simulink model "LKAS_SIL"  (R2018b)
settings: Solver=FixedStepDiscrete  StartTime=0.0  StopTime=90  FixedStep=0.01  MaxStep=0.01  RelTol=1e-3
model workspace (MAT data in the model file):
  LKA_CarWidth = Simulink.Parameter
  LKA_CarWidth.Value = 1.8
  LKA_CarWidth.DataType = 'single'
  LKA_CarWidth.Dimensions = [1 1]
  LKA_SampleTime = Simulink.Parameter
  LKA_SampleTime.Value = 0.01
  LKA_SampleTime.DataType = 'single'
  LKA_SampleTime.Dimensions = [1 1]
  LKA_StrRatio_C = Simulink.Parameter
  LKA_StrRatio_C.Value = 15.3
  LKA_StrRatio_C.DataType = 'single'
  LKA_StrRatio_C.Dimensions = [1 1]
  LKA_Veh2CamL_C = Simulink.Parameter
  LKA_Veh2CamL_C.Value = 1.56
  LKA_Veh2CamL_C.DataType = 'single'
  LKA_Veh2CamL_C.Dimensions = [1 1]
  LKA_Veh2CamW_C = Simulink.Parameter
  LKA_Veh2CamW_C.Value = 0.9
  LKA_Veh2CamW_C.DataType = 'single'
  LKA_Veh2CamW_C.Dimensions = [1 1]
  LKA_WhlBaseL_C = Simulink.Parameter
  LKA_WhlBaseL_C.Value = 2.65
  LKA_WhlBaseL_C.DataType = 'single'
  LKA_WhlBaseL_C.Dimensions = [1 1]
  LL_CompSWA_C = Simulink.Parameter
  LL_CompSWA_C.Value = 0
  LL_CompSWA_C.DataType = 'single'
  LL_CompSWA_C.Dimensions = [1 1]
  LL_CrvtPrvwT_C = Simulink.Parameter
  LL_CrvtPrvwT_C.Value = 0.45
  LL_CrvtPrvwT_C.DataType = 'single'
  LL_CrvtPrvwT_C.Dimensions = [1 1]
  LL_DesDvt_C = Simulink.Parameter
  LL_DesDvt_C.Value = 0.2
  LL_DesDvt_C.DataType = 'single'
  LL_DesDvt_C.Dimensions = [1 1]
  LL_DvtComp_C = Simulink.Parameter
  LL_DvtComp_C.Value = 0
  LL_DvtComp_C.DataType = 'single'
  LL_DvtComp_C.Dimensions = [1 1]
  LL_DvtPrvwT_C = Simulink.Parameter
  LL_DvtPrvwT_C.Value = 0.45
  LL_DvtPrvwT_C.DataType = 'single'
  LL_DvtPrvwT_C.Dimensions = [1 1]
  LL_DvtSpdDet_vDvtSpdMin_C = Simulink.Parameter
  LL_DvtSpdDet_vDvtSpdMin_C.Value = 0
  LL_DvtSpdDet_vDvtSpdMin_C.DataType = 'single'
  LL_DvtSpdDet_vDvtSpdMin_C.Dimensions = [1 1]
  LL_HdAgExT_C = Simulink.Parameter
  LL_HdAgExT_C.Value = 15
  LL_HdAgExT_C.DataType = 'single'
  LL_HdAgExT_C.Dimensions = [1 1]
  LL_HdAgPrvwT_C = Simulink.Parameter
  LL_HdAgPrvwT_C.Value = 0.45
  LL_HdAgPrvwT_C.DataType = 'single'
  LL_HdAgPrvwT_C.Dimensions = [1 1]
  LL_LAccMax_C = Simulink.Parameter
  LL_LAccMax_C.Value = 3
  LL_LAccMax_C.DataType = 'single'
  LL_LAccMax_C.Dimensions = [1 1]
  LL_LAccRMax_C = Simulink.Parameter
  LL_LAccRMax_C.Value = 5
  LL_LAccRMax_C.DataType = 'single'
  LL_LAccRMax_C.Dimensions = [1 1]
  LL_LDWS_SUPPRESS_HEADING = Simulink.Parameter
  LL_LDWS_SUPPRESS_HEADING.Value = 2
  LL_LDWS_SUPPRESS_HEADING.DataType = 'single'
  LL_LDWS_SUPPRESS_HEADING.Dimensions = [1 1]
  LL_LDW_EarliestWarnLine_C = Simulink.Parameter
  LL_LDW_EarliestWarnLine_C.Value = 0.3
  LL_LDW_EarliestWarnLine_C.DataType = 'single'
  LL_LDW_EarliestWarnLine_C.Dimensions = [1 1]
  LL_LDW_LatestWarnLine_C = Simulink.Parameter
  LL_LDW_LatestWarnLine_C.Value = -0.4
  LL_LDW_LatestWarnLine_C.DataType = 'single'
  LL_LDW_LatestWarnLine_C.Dimensions = [1 1]
  LL_LFClb_TFC_DiffCtlBalance = Simulink.Parameter
  LL_LFClb_TFC_DiffCtlBalance.Value = 0
  LL_LFClb_TFC_DiffCtlBalance.DataType = 'single'
  LL_LFClb_TFC_DiffCtlBalance.Dimensions = [1 1]
  LL_LFClb_TFC_DiffCtrlMaxSWA = Simulink.Parameter
  LL_LFClb_TFC_DiffCtrlMaxSWA.Value = 20
  LL_LFClb_TFC_DiffCtrlMaxSWA.DataType = 'single'
  LL_LFClb_TFC_DiffCtrlMaxSWA.Dimensions = [1 1]
  LL_LFClb_TFC_DiffCtrlRatio = Simulink.Parameter
  LL_LFClb_TFC_DiffCtrlRatio.Value = 400
  LL_LFClb_TFC_DiffCtrlRatio.DataType = 'single'
  LL_LFClb_TFC_DiffCtrlRatio.Dimensions = [1 1]
  LL_LFClb_TFC_FfCtlRatio_C = Simulink.Parameter
  LL_LFClb_TFC_FfCtlRatio_C.Value = 1
  LL_LFClb_TFC_FfCtlRatio_C.DataType = 'single'
  LL_LFClb_TFC_FfCtlRatio_C.Dimensions = [1 1]
  LL_LFClb_TFC_facmGainLutGain1_C = Simulink.Parameter
  LL_LFClb_TFC_facmGainLutGain1_C.Value = 40
  LL_LFClb_TFC_facmGainLutGain1_C.DataType = 'single'
  LL_LFClb_TFC_facmGainLutGain1_C.Dimensions = [1 1]
  LL_LFClb_TFC_facmGainLutGain2_C = Simulink.Parameter
  LL_LFClb_TFC_facmGainLutGain2_C.Value = 40
  LL_LFClb_TFC_facmGainLutGain2_C.DataType = 'single'
  LL_LFClb_TFC_facmGainLutGain2_C.Dimensions = [1 1]
  LL_LFClb_TFC_facmIntegRatio = Simulink.Parameter
  LL_LFClb_TFC_facmIntegRatio.Value = 0.002
  LL_LFClb_TFC_facmIntegRatio.DataType = 'single'
  LL_LFClb_TFC_facmIntegRatio.Dimensions = [1 1]
  LL_LFClb_TFC_facmKlat_C = Simulink.Parameter
  LL_LFClb_TFC_facmKlat_C.Value = -9
  LL_LFClb_TFC_facmKlat_C.DataType = 'single'
  LL_LFClb_TFC_facmKlat_C.Dimensions = [1 1]
  LL_LFClb_TFC_phiIntegCtlMaxSWA_C = Simulink.Parameter
  LL_LFClb_TFC_phiIntegCtlMaxSWA_C.Value = 5
  LL_LFClb_TFC_phiIntegCtlMaxSWA_C.DataType = 'single'
  LL_LFClb_TFC_phiIntegCtlMaxSWA_C.Dimensions = [1 1]
  LL_LFClb_TFC_tiKlatPrvwT_C = Simulink.Parameter
  LL_LFClb_TFC_tiKlatPrvwT_C.Value = 2
  LL_LFClb_TFC_tiKlatPrvwT_C.DataType = 'single'
  LL_LFClb_TFC_tiKlatPrvwT_C.Dimensions = [1 1]
  LL_LFClb_TFC_vGainLutVehSpdLwr_C = Simulink.Parameter
  LL_LFClb_TFC_vGainLutVehSpdLwr_C.Value = 60
  LL_LFClb_TFC_vGainLutVehSpdLwr_C.DataType = 'single'
  LL_LFClb_TFC_vGainLutVehSpdLwr_C.Dimensions = [1 1]
  LL_LFClb_TFC_vGainLutVehSpdUpr_C = Simulink.Parameter
  LL_LFClb_TFC_vGainLutVehSpdUpr_C.Value = 120
  LL_LFClb_TFC_vGainLutVehSpdUpr_C.DataType = 'single'
  LL_LFClb_TFC_vGainLutVehSpdUpr_C.Dimensions = [1 1]
  LL_LKAExPrcs_ExitC0Dvt = Simulink.Parameter
  LL_LKAExPrcs_ExitC0Dvt.Value = 0.01
  LL_LKAExPrcs_ExitC0Dvt.DataType = 'single'
  LL_LKAExPrcs_ExitC0Dvt.Dimensions = [1 1]
  LL_LKAExPrcs_ExitC0Swt = Simulink.Parameter
  LL_LKAExPrcs_ExitC0Swt.Value = 1
  LL_LKAExPrcs_ExitC0Swt.DataType = 'single'
  LL_LKAExPrcs_ExitC0Swt.Dimensions = [1 1]
  LL_LKAExPrcs_tiExitTime1 = Simulink.Parameter
  LL_LKAExPrcs_tiExitTime1.Value = 8
  LL_LKAExPrcs_tiExitTime1.DataType = 'single'
  LL_LKAExPrcs_tiExitTime1.Dimensions = [1 1]
  LL_LKAExPrcs_tiExitTime2 = Simulink.Parameter
  LL_LKAExPrcs_tiExitTime2.Value = 4
  LL_LKAExPrcs_tiExitTime2.DataType = 'single'
  LL_LKAExPrcs_tiExitTime2.Dimensions = [1 1]
  LL_LKAExPrcs_tiExitTime3 = Simulink.Parameter
  LL_LKAExPrcs_tiExitTime3.Value = 0.2
  LL_LKAExPrcs_tiExitTime3.DataType = 'single'
  LL_LKAExPrcs_tiExitTime3.Dimensions = [1 1]
  LL_LKASWASyn_M0 = Simulink.Parameter
  LL_LKASWASyn_M0.Value = 0.4
  LL_LKASWASyn_M0.DataType = 'single'
  LL_LKASWASyn_M0.Dimensions = [1 1]
  LL_LKASWASyn_M1 = Simulink.Parameter
  LL_LKASWASyn_M1.Value = 0.8
  LL_LKASWASyn_M1.DataType = 'single'
  LL_LKASWASyn_M1.Dimensions = [1 1]
  LL_LKASWASyn_M2 = Simulink.Parameter
  LL_LKASWASyn_M2.Value = 0.3
  LL_LKASWASyn_M2.DataType = 'single'
  LL_LKASWASyn_M2.Dimensions = [1 1]
  LL_LKASWASyn_M3K = Simulink.Parameter
  LL_LKASWASyn_M3K.Value = 0.2
  LL_LKASWASyn_M3K.DataType = 'single'
  LL_LKASWASyn_M3K.Dimensions = [1 1]
  LL_LKASWASyn_SWAaddMax = Simulink.Parameter
  LL_LKASWASyn_SWAaddMax.Value = 8
  LL_LKASWASyn_SWAaddMax.DataType = 'single'
  LL_LKASWASyn_SWAaddMax.Dimensions = [1 1]
  LL_LKASWASyn_T2 = Simulink.Parameter
  LL_LKASWASyn_T2.Value = 4
  LL_LKASWASyn_T2.DataType = 'single'
  LL_LKASWASyn_T2.Dimensions = [1 1]
  LL_LKASWASyn_TrqMax = Simulink.Parameter
  LL_LKASWASyn_TrqMax.Value = 1.5
  LL_LKASWASyn_TrqMax.DataType = 'single'
  LL_LKASWASyn_TrqMax.Dimensions = [1 1]
  LL_LKASWASyn_TrqSwaAddSwt = Simulink.Parameter
  LL_LKASWASyn_TrqSwaAddSwt.Value = 0
  LL_LKASWASyn_TrqSwaAddSwt.DataType = 'single'
  LL_LKASWASyn_TrqSwaAddSwt.Dimensions = [1 1]
  LL_LKASWASyn_TrqSwaRateDiff = Simulink.Parameter
  LL_LKASWASyn_TrqSwaRateDiff.Value = -0.2
  LL_LKASWASyn_TrqSwaRateDiff.DataType = 'single'
  LL_LKASWASyn_TrqSwaRateDiff.Dimensions = [1 1]
  LL_LKASWASyn_tiTrqSwaRtTime = Simulink.Parameter
  LL_LKASWASyn_tiTrqSwaRtTime.Value = 0.2
  LL_LKASWASyn_tiTrqSwaRtTime.DataType = 'single'
  LL_LKASWASyn_tiTrqSwaRtTime.Dimensions = [1 1]
  LL_LKASWASyn_tiTrqSwaTime = Simulink.Parameter
  LL_LKASWASyn_tiTrqSwaTime.Value = 0.3
  LL_LKASWASyn_tiTrqSwaTime.DataType = 'single'
  LL_LKASWASyn_tiTrqSwaTime.Dimensions = [1 1]
  LL_LKAS_OUT_OF_CONTROL_LAT_VEL = Simulink.Parameter
  LL_LKAS_OUT_OF_CONTROL_LAT_VEL.Value = 1.5
  LL_LKAS_OUT_OF_CONTROL_LAT_VEL.DataType = 'single'
  LL_LKAS_OUT_OF_CONTROL_LAT_VEL.Dimensions = [1 1]
  LL_LKAS_OUT_OF_CONTROL_TTLC = Simulink.Parameter
  LL_LKAS_OUT_OF_CONTROL_TTLC.Value = 0.3
  LL_LKAS_OUT_OF_CONTROL_TTLC.DataType = 'single'
  LL_LKAS_OUT_OF_CONTROL_TTLC.Dimensions = [1 1]
  LL_LKA_EarliestWarnLine_C = Simulink.Parameter
  LL_LKA_EarliestWarnLine_C.Value = 0.3
  LL_LKA_EarliestWarnLine_C.DataType = 'single'
  LL_LKA_EarliestWarnLine_C.Dimensions = [1 1]
  LL_LKA_LatestWarnLine_C = Simulink.Parameter
  LL_LKA_LatestWarnLine_C.Value = -0.5
  LL_LKA_LatestWarnLine_C.DataType = 'single'
  LL_LKA_LatestWarnLine_C.Dimensions = [1 1]
  LL_LSpdCompT_C = Simulink.Parameter
  LL_LSpdCompT_C.Value = 0.4
  LL_LSpdCompT_C.DataType = 'single'
  LL_LSpdCompT_C.Dimensions = [1 1]
  LL_MAX_DELAY_EPSSTAR_TIME = Simulink.Parameter
  LL_MAX_DELAY_EPSSTAR_TIME.Value = 0.5
  LL_MAX_DELAY_EPSSTAR_TIME.DataType = 'single'
  LL_MAX_DELAY_EPSSTAR_TIME.Dimensions = [1 1]
  LL_MAX_DRIVER_TORQUE_DISABLE = Simulink.Parameter
  LL_MAX_DRIVER_TORQUE_DISABLE.Value = 2.25
  LL_MAX_DRIVER_TORQUE_DISABLE.DataType = 'single'
  LL_MAX_DRIVER_TORQUE_DISABLE.Dimensions = [1 1]
  LL_MAX_DRIVER_TORQUE_ENABLE = Simulink.Parameter
  LL_MAX_DRIVER_TORQUE_ENABLE.Value = 3
  LL_MAX_DRIVER_TORQUE_ENABLE.DataType = 'single'
  LL_MAX_DRIVER_TORQUE_ENABLE.Dimensions = [1 1]
  LL_MAX_LANE_WIDTH_DISABLE = Simulink.Parameter
  LL_MAX_LANE_WIDTH_DISABLE.Value = 5.5
  LL_MAX_LANE_WIDTH_DISABLE.DataType = 'single'
  LL_MAX_LANE_WIDTH_DISABLE.Dimensions = [1 1]
  LL_MAX_LANE_WIDTH_ENABLE = Simulink.Parameter
  LL_MAX_LANE_WIDTH_ENABLE.Value = 5.4
  LL_MAX_LANE_WIDTH_ENABLE.DataType = 'single'
  LL_MAX_LANE_WIDTH_ENABLE.Dimensions = [1 1]
  LL_MAX_LAT_ACC_DISABLE = Simulink.Parameter
  LL_MAX_LAT_ACC_DISABLE.Value = 3.5
  LL_MAX_LAT_ACC_DISABLE.DataType = 'single'
  LL_MAX_LAT_ACC_DISABLE.Dimensions = [1 1]
  LL_MAX_LAT_ACC_ENABLE = Simulink.Parameter
  LL_MAX_LAT_ACC_ENABLE.Value = 3
  LL_MAX_LAT_ACC_ENABLE.DataType = 'single'
  LL_MAX_LAT_ACC_ENABLE.Dimensions = [1 1]
  LL_MAX_LDWS_SPEED_DISABLE = Simulink.Parameter
  LL_MAX_LDWS_SPEED_DISABLE.Value = 150
  LL_MAX_LDWS_SPEED_DISABLE.DataType = 'single'
  LL_MAX_LDWS_SPEED_DISABLE.Dimensions = [1 1]
  LL_MAX_LDWS_SPEED_ENABLE = Simulink.Parameter
  LL_MAX_LDWS_SPEED_ENABLE.Value = 140
  LL_MAX_LDWS_SPEED_ENABLE.DataType = 'single'
  LL_MAX_LDWS_SPEED_ENABLE.Dimensions = [1 1]
  LL_MAX_LKAS_SPEED_DISABLE = Simulink.Parameter
  LL_MAX_LKAS_SPEED_DISABLE.Value = 150
  LL_MAX_LKAS_SPEED_DISABLE.DataType = 'single'
  LL_MAX_LKAS_SPEED_DISABLE.Dimensions = [1 1]
  LL_MAX_LKAS_SPEED_ENABLE = Simulink.Parameter
  LL_MAX_LKAS_SPEED_ENABLE.Value = 140
  LL_MAX_LKAS_SPEED_ENABLE.DataType = 'single'
  LL_MAX_LKAS_SPEED_ENABLE.Dimensions = [1 1]
  LL_MAX_LONG_ACC_DISABLE = Simulink.Parameter
  LL_MAX_LONG_ACC_DISABLE.Value = 3.5
  LL_MAX_LONG_ACC_DISABLE.DataType = 'single'
  LL_MAX_LONG_ACC_DISABLE.Dimensions = [1 1]
  LL_MAX_LONG_ACC_ENABLE = Simulink.Parameter
  LL_MAX_LONG_ACC_ENABLE.Value = 3
  LL_MAX_LONG_ACC_ENABLE.DataType = 'single'
  LL_MAX_LONG_ACC_ENABLE.Dimensions = [1 1]
  LL_MAX_LONG_DECEL_DISABLE = Simulink.Parameter
  LL_MAX_LONG_DECEL_DISABLE.Value = 2.5
  LL_MAX_LONG_DECEL_DISABLE.DataType = 'single'
  LL_MAX_LONG_DECEL_DISABLE.Dimensions = [1 1]
  LL_MAX_LONG_DECEL_ENABLE = Simulink.Parameter
  LL_MAX_LONG_DECEL_ENABLE.Value = 2
  LL_MAX_LONG_DECEL_ENABLE.DataType = 'single'
  LL_MAX_LONG_DECEL_ENABLE.Dimensions = [1 1]
  LL_MAX_STEER_ANGLE_DISABLE = Simulink.Parameter
  LL_MAX_STEER_ANGLE_DISABLE.Value = 70
  LL_MAX_STEER_ANGLE_DISABLE.DataType = 'single'
  LL_MAX_STEER_ANGLE_DISABLE.Dimensions = [1 1]
  LL_MAX_STEER_ANGLE_ENABLE = Simulink.Parameter
  LL_MAX_STEER_ANGLE_ENABLE.Value = 60
  LL_MAX_STEER_ANGLE_ENABLE.DataType = 'single'
  LL_MAX_STEER_ANGLE_ENABLE.Dimensions = [1 1]
  LL_MAX_STEER_SPEED_DISABLE = Simulink.Parameter
  LL_MAX_STEER_SPEED_DISABLE.Value = 5000
  LL_MAX_STEER_SPEED_DISABLE.DataType = 'single'
  LL_MAX_STEER_SPEED_DISABLE.Dimensions = [1 1]
  LL_MAX_STEER_SPEED_ENABLE = Simulink.Parameter
  LL_MAX_STEER_SPEED_ENABLE.Value = 5000
  LL_MAX_STEER_SPEED_ENABLE.DataType = 'single'
  LL_MAX_STEER_SPEED_ENABLE.Dimensions = [1 1]
  LL_MAX_SYSTEM_CURVATURE_DISABLE = Simulink.Parameter
  LL_MAX_SYSTEM_CURVATURE_DISABLE.Value = 0.0055
  LL_MAX_SYSTEM_CURVATURE_DISABLE.DataType = 'single'
  LL_MAX_SYSTEM_CURVATURE_DISABLE.Dimensions = [1 1]
  LL_MAX_SYSTEM_CURVATURE_ENABLE = Simulink.Parameter
  LL_MAX_SYSTEM_CURVATURE_ENABLE.Value = 0.0045
  LL_MAX_SYSTEM_CURVATURE_ENABLE.DataType = 'single'
  LL_MAX_SYSTEM_CURVATURE_ENABLE.Dimensions = [1 1]
  LL_MIN_LANE_WIDTH_DISABLE = Simulink.Parameter
  LL_MIN_LANE_WIDTH_DISABLE.Value = 2.4
  LL_MIN_LANE_WIDTH_DISABLE.DataType = 'single'
  LL_MIN_LANE_WIDTH_DISABLE.Dimensions = [1 1]
  LL_MIN_LANE_WIDTH_ENABLE = Simulink.Parameter
  LL_MIN_LANE_WIDTH_ENABLE.Value = 2.5
  LL_MIN_LANE_WIDTH_ENABLE.DataType = 'single'
  LL_MIN_LANE_WIDTH_ENABLE.Dimensions = [1 1]
  LL_MIN_LKAS_SPEED_DISABLE = Simulink.Parameter
  LL_MIN_LKAS_SPEED_DISABLE.Value = 55
  LL_MIN_LKAS_SPEED_DISABLE.DataType = 'single'
  LL_MIN_LKAS_SPEED_DISABLE.Dimensions = [1 1]
  LL_MIN_LKAS_SPEED_ENABLE = Simulink.Parameter
  LL_MIN_LKAS_SPEED_ENABLE.Value = 60
  LL_MIN_LKAS_SPEED_ENABLE.DataType = 'single'
  LL_MIN_LKAS_SPEED_ENABLE.Dimensions = [1 1]
  LL_Max_LDWS_Warning_Time = Simulink.Parameter
  LL_Max_LDWS_Warning_Time.Value = 5
  LL_Max_LDWS_Warning_Time.DataType = 'single'
  LL_Max_LDWS_Warning_Time.Dimensions = [1 1]
  LL_NomTAhd_C = Simulink.Parameter
  LL_NomTAhd_C.Value = 0.2
  LL_NomTAhd_C.DataType = 'single'
  LL_NomTAhd_C.Dimensions = [1 1]
  LL_ThresDet_lDvtThresLwrLDW = Simulink.Parameter
  LL_ThresDet_lDvtThresLwrLDW.Value = 0.15
  LL_ThresDet_lDvtThresLwrLDW.DataType = 'single'
  LL_ThresDet_lDvtThresLwrLDW.Dimensions = [1 1]
  LL_ThresDet_lDvtThresLwrLKA = Simulink.Parameter
  LL_ThresDet_lDvtThresLwrLKA.Value = 0.3
  LL_ThresDet_lDvtThresLwrLKA.DataType = 'single'
  LL_ThresDet_lDvtThresLwrLKA.Dimensions = [1 1]
  LL_ThresDet_lDvtThresUprLDW = Simulink.Parameter
  LL_ThresDet_lDvtThresUprLDW.Value = 0.3
  LL_ThresDet_lDvtThresUprLDW.DataType = 'single'
  LL_ThresDet_lDvtThresUprLDW.Dimensions = [1 1]
  LL_ThresDet_lDvtThresUprLKA = Simulink.Parameter
  LL_ThresDet_lDvtThresUprLKA.Value = 0.6
  LL_ThresDet_lDvtThresUprLKA.DataType = 'single'
  LL_ThresDet_lDvtThresUprLKA.Dimensions = [1 1]
  LL_ThresDet_tiTTLCThresLDW = Simulink.Parameter
  LL_ThresDet_tiTTLCThresLDW.Value = 0.75
  LL_ThresDet_tiTTLCThresLDW.DataType = 'single'
  LL_ThresDet_tiTTLCThresLDW.Dimensions = [1 1]
  LL_ThresDet_tiTTLCThresLKA = Simulink.Parameter
  LL_ThresDet_tiTTLCThresLKA.Value = 1.5
  LL_ThresDet_tiTTLCThresLKA.DataType = 'single'
  LL_ThresDet_tiTTLCThresLKA.Dimensions = [1 1]
  LL_TkOvStChk_tiTDelTime = Simulink.Parameter
  LL_TkOvStChk_tiTDelTime.Value = 2
  LL_TkOvStChk_tiTDelTime.DataType = 'single'
  LL_TkOvStChk_tiTDelTime.Dimensions = [1 1]
  LL_TkOvStChk_tiTrqChkT = Simulink.Parameter
  LL_TkOvStChk_tiTrqChkT.Value = 0.1
  LL_TkOvStChk_tiTrqChkT.DataType = 'single'
  LL_TkOvStChk_tiTrqChkT.Dimensions = [1 1]
  LL_lStpLngth_C = Simulink.Parameter
  LL_lStpLngth_C.Value = 5
  LL_lStpLngth_C.DataType = 'single'
  LL_lStpLngth_C.Dimensions = [1 1]
  ob_LKA_Version = Simulink.Signal
  ob_LKA_Version.DataType = 'single'
  ob_LKA_Version.Dimensions = -1
  ob_LKA_Version.DimensionsMode = 'auto'
  ob_LKA_Version.Complexity = 'auto'
  ob_LKA_Version.SampleTime = -1
  ob_LKA_Version.SamplingMode = 'auto'
undefined symbols (not defined in the file or in its folder): LKA_CarWidth, LKA_SampleTime, LKA_StrRatio_C, LKA_Veh2CamL_C, LKA_Veh2CamW_C, LKA_WhlBaseL_C, LL_CompSWA_C, LL_CrvtPrvwT_C, LL_DesDvt_C, LL_DvtComp_C, LL_DvtPrvwT_C, LL_DvtSpdDet_vDvtSpdMin_C, LL_HdAgExT_C, LL_HdAgPrvwT_C, LL_LAccMax_C, LL_LAccRMax_C, LL_LDW_EarliestWarnLine_C, LL_LDW_LatestWarnLine_C, LL_LDWS_SUPPRESS_HEADING, LL_LFClb_TFC_DiffCtlBalance, LL_LFClb_TFC_DiffCtrlMaxSWA, LL_LFClb_TFC_DiffCtrlRatio, LL_LFClb_TFC_facmGainLutGain1_C, LL_LFClb_TFC_facmGainLutGain2_C, LL_LFClb_TFC_facmIntegRatio, LL_LFClb_TFC_facmKlat_C, LL_LFClb_TFC_FfCtlRatio_C, LL_LFClb_TFC_phiIntegCtlMaxSWA_C, LL_LFClb_TFC_tiKlatPrvwT_C, LL_LFClb_TFC_vGainLutVehSpdLwr_C, LL_LFClb_TFC_vGainLutVehSpdUpr_C, LL_LKA_EarliestWarnLine_C, LL_LKA_LatestWarnLine_C, LL_LKAExPrcs_ExitC0Dvt, LL_LKAExPrcs_ExitC0Swt, LL_LKAExPrcs_tiExitTime1, LL_LKAExPrcs_tiExitTime2, LL_LKAExPrcs_tiExitTime3, LL_LKAS_OUT_OF_CONTROL_LAT_VEL, LL_LKAS_OUT_OF_CONTROL_TTLC, LL_LKASWASyn_M0, LL_LKASWASyn_M1, LL_LKASWASyn_M2, LL_LKASWASyn_M3K, LL_LKASWASyn_SWAaddMax, LL_LKASWASyn_T2, LL_LKASWASyn_tiTrqSwaRtTime, LL_LKASWASyn_tiTrqSwaTime, LL_LKASWASyn_TrqMax, LL_LKASWASyn_TrqSwaAddSwt, LL_LKASWASyn_TrqSwaRateDiff, LL_LSpdCompT_C, LL_lStpLngth_C, LL_MAX_DELAY_EPSSTAR_TIME, LL_MAX_DRIVER_TORQUE_DISABLE, LL_MAX_DRIVER_TORQUE_ENABLE, LL_MAX_LANE_WIDTH_DISABLE, LL_MAX_LANE_WIDTH_ENABLE, LL_MAX_LAT_ACC_DISABLE, LL_MAX_LAT_ACC_ENABLE ... (+29)
libraries: simulink x134, dspstat3 x3, simulink_extras x1
(part 1 of 13)
settings Model: SimulationMode=software-in-the-loop (sil)  Creator=hejr  LastModifiedBy=hejr
settings DataIOCC: ExternalInput=[Time,GW_550_PSA1__LKA_main_switch,GW_550_PSA1__LC_Mode,EPS_495_PSA1__State_of_EPS_for_LKA_function,EPS_495_PSA1__Steering_wheel_torque,ESC_3CD_PSA1__Lateral_acceleration,ESC_3CD_PSA1__Yaw_speed,ESC_38D_PSA1__Vehicle_speed_of_wheelsensor,GW_32D_PSA1__ACCEL_LONGI_CALIB,ESC_3CD_PSA1__TMC_pressure,EPS_305_PSA1__Steering_wheel_angle,EPS_305_PSA1__Steering_wheel_rotation_speed,GW_452_PSA1__BCM_Status_Indicator,GW_349_PSA1__TCU_Gear_lever_position,Video_Lane_Left_A__C3_5FA,Video_Lane_Left_A__C2_5FA,Video_Lane_Left_A__C1_5FA,Video_Lane_Left_A__C0_5FA,Video_Lane_Left_A__Quality_5FA,Video_Lane_Left_A__Line_Type_5FA,Video_Lane_Left_B__View_Range_5FC,Video_Lane_Left_B__TLC_5FC,Video_Lane_Right_A__C3_5FD,Video_Lane_Right_A__C2_5FD,Video_Lane_Right_A__C1_5FD,Video_Lane_Right_A__C0_5FD,Video_Lane_Right_A__Quality_5FD,Video_Lane_Right_A__Line_Type_5FD,Video_Lane_Right_B__View_Range_5FF,Video_Lane_Right_B__TLC_5FF,Video_Lane_Left_A__C0_5FA,Video_Lane_Left_A__C1_5FA,Video_Lane_Left_A__C2_5FA,Video_Lane_Left_A__C3_5FA,Video_Lane_Left_B__View_Range_5FC,Video_Lane_Left_A__Quality_5FA,Video_Lane_Left_A__Line_Type_5FA,Video_Lane_Left_B__TLC_5FC,Video_Lane_Right_A__C0_5FD,Video_Lane_Right_A__C1_5FD,Video_Lane_Right_A__C2_5FD,Video_Lane_Right_A__C3_5FD,Video_Lane_Right_B__View_Range_5FF,Video_Lane_Right_A__Quality_5FD,Video_Lane_Right_A__Line_Type_5FD,Video_Lane_Right_B__TLC_5FF,ADAS_541_PSA1__LDW_Flag,ADAS_541_PSA1__Vehicle_Lane_Display,ADAS_3F2_PSA1__Column_angle_setpoint3F2,ADAS_3F2_PSA1__Permit_to_know_if_LKA_or_LPA3F2]  LoadExternalInput=on  SaveFormat=StructureWithTime  SaveOutput=off  SignalLoggingName=logsOut
settings OptimizationCC: DefaultParameterBehavior=Inlined  DefaultUnderspecifiedDataType=single  EnhancedBackFolding=on  PassReuseOutputArgsAs=Individual arguments  ZeroExternalMemoryAtStartup=off  ZeroInternalMemoryAtStartup=off  OptimizeBlockOrder=speed  DifferentSizesBufferReuse=on  OptimizationCustomize=off
settings DebuggingCC: ParameterTunabilityLossMsg=error
settings SFSimCC: MATLABDynamicMemAlloc=off
settings RTWCC: SystemTargetFile=autosar.tlc  TemplateMakefile=ert_default_tmf  Description=AUTOSAR  GenerateReport=on  Toolchain=MinGW64 | gmake (64-bit Windows)  IncludeHyperlinkInReport=on  LaunchReport=on  GenerateTraceInfo=on  GenerateTraceReport=on  GenerateTraceReportSl=on  GenerateTraceReportSf=on  GenerateTraceReportEml=on
settings CodeAppCC: ForceParamTrailComments=on  IgnoreCustomStorageClasses=off  OperatorAnnotations=on  SimulinkDataObjDesc=on  SFDataObjDesc=on  InsertBlockDesc=on
settings STFCustomTargetCC: TargetLangStandard=C99 (ISO)  MultiwordLength=256  ParMdlRefBuildCompliant=on  CompOptLevelCompliant=on  IncludeMdlTerminateFcn=off  CombineOutputUpdateFcns=on  SuppressErrorStatus=on  ERTCustomFileBanners=on  SupportNonFinite=off  SupportComplex=off  SupportContinuousTime=off  SupportNonInlinedSFcns=off  RemoveResetFunc=on  MATLABClassNameForMDSCustomization=Simulink.SoftwareTarget.ERTCustomization  AutosarCompliant=on  UseToolchainInfoCompliant=on  LookupTableObjectStructAxisOrder=2,1,3,4,...  LUTObjectStructOrderEvenSpacing=Size,Table,Breakpoints  SystemTargetFile=autosar.tlc
settings ERTTargetCC: TargetLangStandard=C99 (ISO)  ConcurrentExecutionCompliant=off  IncludeMdlTerminateFcn=off  SuppressErrorStatus=on  SupportNonFinite=off  SupportComplex=off  ModelStepFunctionPrototypeControlCompliant=off  CPPClassGenCompliant=off  AutosarCompliant=on  LookupTableObjectStructAxisOrder=2,1,3,4,...  LUTObjectStructOrderEvenSpacing=Size,Table,Breakpoints  InlinedParameterPlacement=NonHierarchical  ERTCustomFileTemplate=example_file_process.tlc

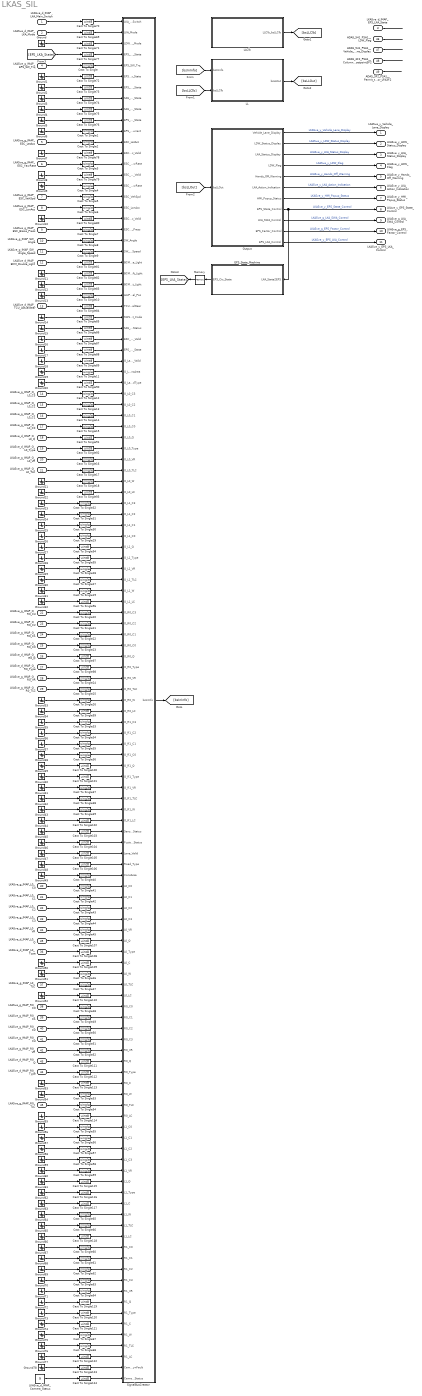
== system LKAS_SIL ==
  LKASve_d_IMAP_LKA_Main_Switch : Inport  OutDataTypeStr=double
  LKASve_d_IMAP_LKA_Mode : Inport  Port=2  OutDataTypeStr=double
  LKASve_d_IMAP_EPS_LKA_State : Inport  Port=3  OutDataTypeStr=double
  LKASve_g_IMAP_EPS_SW_Trq : Inport  Port=4  OutDataTypeStr=double
  LKASve_g_IMAP_ESC_LatAcc : Inport  Port=5  OutDataTypeStr=double
  LKASve_g_IMAP_ESC_YawRate : Inport  Port=6  OutDataTypeStr=double
  LKASve_g_IMAP_ESC_VehSpd : Inport  Port=7  OutDataTypeStr=double
  LKASve_g_IMAP_ESC_LonAcc : Inport  Port=8  OutDataTypeStr=double
  LKASve_g_IMAP_ESC_Brake_Press : Inport  Port=9  OutDataTypeStr=double
  LKASve_g_IMAP_SW_Angle : Inport  Port=10  OutDataTypeStr=double
  LKASve_g_IMAP_SW_Angle_Speed : Inport  Port=11  OutDataTypeStr=double
  LKASve_d_IMAP_BCM_Double_Light : Inport  Port=12  OutDataTypeStr=double
  LKASve_d_IMAP_TCU_ActualGear : Inport  Port=13  OutDataTypeStr=double
  LKASve_g_IMAP_O_L0_C3 : Inport  Port=14  OutDataTypeStr=double
  LKASve_g_IMAP_O_L0_C2 : Inport  Port=15  OutDataTypeStr=double
  LKASve_g_IMAP_O_L0_C1 : Inport  Port=16  OutDataTypeStr=double
  LKASve_g_IMAP_O_L0_C0 : Inport  Port=17  OutDataTypeStr=double
  LKASve_d_IMAP_O_L0_Q : Inport  Port=18  OutDataTypeStr=double
  LKASve_d_IMAP_O_L0_Type : Inport  Port=19  OutDataTypeStr=double
  LKASve_g_IMAP_O_L0_VR : Inport  Port=20  OutDataTypeStr=double
  LKASve_g_IMAP_O_L0_TLC : Inport  Port=21  OutDataTypeStr=double
  LKASve_g_IMAP_O_R0_C3 : Inport  Port=22  OutDataTypeStr=double
  LKASve_g_IMAP_O_R0_C2 : Inport  Port=23  OutDataTypeStr=double
  LKASve_g_IMAP_O_R0_C1 : Inport  Port=24  OutDataTypeStr=double
  LKASve_g_IMAP_O_R0_C0 : Inport  Port=25  OutDataTypeStr=double
  LKASve_d_IMAP_O_R0_Q : Inport  Port=26  OutDataTypeStr=double
  LKASve_d_IMAP_O_R0_Type : Inport  Port=27  OutDataTypeStr=double
  LKASve_g_IMAP_O_R0_VR : Inport  Port=28  OutDataTypeStr=double
  LKASve_g_IMAP_O_R0_TLC : Inport  Port=29  OutDataTypeStr=double
  LKASve_g_IMAP_L0_C0 : Inport  Port=30  OutDataTypeStr=double
  LKASve_g_IMAP_L0_C1 : Inport  Port=31  OutDataTypeStr=double
  LKASve_g_IMAP_L0_C2 : Inport  Port=32  OutDataTypeStr=double
  LKASve_g_IMAP_L0_C3 : Inport  Port=33  OutDataTypeStr=double
  LKASve_g_IMAP_L0_VR : Inport  Port=34  OutDataTypeStr=double
  LKASve_d_IMAP_L0_Q : Inport  Port=35  OutDataTypeStr=double
  LKASve_d_IMAP_L0_Type : Inport  Port=36  OutDataTypeStr=double
  LKASve_g_IMAP_L0_TLC : Inport  Port=37  OutDataTypeStr=double
  LKASve_g_IMAP_R0_C0 : Inport  Port=38  OutDataTypeStr=double
  LKASve_g_IMAP_R0_C1 : Inport  Port=39  OutDataTypeStr=double
  LKASve_g_IMAP_R0_C2 : Inport  Port=40  OutDataTypeStr=double
  LKASve_g_IMAP_R0_C3 : Inport  Port=41  OutDataTypeStr=double
  LKASve_g_IMAP_R0_VR : Inport  Port=42  OutDataTypeStr=double
  LKASve_d_IMAP_R0_Q : Inport  Port=43  OutDataTypeStr=double
  LKASve_d_IMAP_R0_Type : Inport  Port=44  OutDataTypeStr=double
  LKASve_g_IMAP_R0_TLC : Inport  Port=45  OutDataTypeStr=double
  ADAS_541_PSA1__LDW_Flag : Inport  Port=46  OutDataTypeStr=double
  ADAS_541_PSA1__Vehicle_Lane_Display : Inport  Port=47  OutDataTypeStr=double
  ADAS_3F2_PSA1__Column_angle_setpoint3F2 : Inport  Port=48  OutDataTypeStr=double
  ADAS_3F2_PSA1__Permit_to_know_if_LKA_or_LPA3F2 : Inport  Port=49  OutDataTypeStr=double
  Cast To Single{,1..68} (69 alike) : DataTypeConversion  OutDataTypeStr=single
  Cast To Single{69..124} (56 alike) : DataTypeConversion  OutDataTypeStr=uint8
  EPS_State_Mashine : Subsystem
  Ground{,1..78} (79 alike) : Ground
  LKASve_d_IMAP_Camera_Status : Constant  Value=9  OutDataTypeStr=uint8
  LL : Subsystem  TreatAsAtomicUnit=on
  LLClb : Subsystem
  Memory : Memory
  Output : Subsystem
  SignalBusCreator : Subsystem
  LKASve_y_Vehicle_Lane_Display : Outport
  LKASve_y_LDW_Status_Display : Outport  Port=2  SignalName=LKASve_y_LDW_Status_Display
  LKASve_y_LKA_Status_Display : Outport  Port=3
  LKASve_y_LDW_Flag : Outport  Port=4
  LKASve_y_Hands_Off_Warning : Outport  Port=5
  LKASve_y_LKA_Action_Indication : Outport  Port=6
  LKASve_y_HMI_Popup_Status : Outport  Port=7
  LKAve_y_EPS_State_Control : Outport  Port=8
  LKASve_g_LKA_SWA_Control : Outport  Port=9
  LKASve_g_EPS_Factor_Control : Outport  Port=10
  LKASve_y_EPS_LKA_Control : Outport  Port=11
  wires:
  LKASve_g_IMAP_O_L0_C1/1 -> Cast To Single14/1
  LKASve_g_IMAP_O_L0_TLC/1 -> Cast To Single17/1
  Ground61/1 -> Cast To Single115/1
  Cast To Single4/1 -> SignalBusCreator/16(ESC_UnYawRate)
  LKASve_d_IMAP_O_L0_Type/1 -> Cast To Single92/1
  Cast To Single107/1 -> SignalBusCreator/85(L0_Q)
  Cast To Single16/1 -> SignalBusCreator/41(O_L0_VR)
  Cast To Single73/1 -> SignalBusCreator/7(EPS_Trq_State)
  Cast To Single34/1 -> SignalBusCreator/66(O_R1_C2)
  Cast To Single80/1 -> SignalBusCreator/19(ESC_LonAcc_Valid)
  Ground31/1 -> Cast To Single19/1
  Cast To Single22/1 -> SignalBusCreator/57(O_R0_C1)
  Cast To Single77/1 -> SignalBusCreator/4(EPS_LKA_State)
  Cast To Single60/1 -> SignalBusCreator/113(R1_C0)
  Ground70/1 -> Cast To Single63/1
  Ground75/1 -> Cast To Single67/1
  Cast To Single49/1 -> SignalBusCreator/92(R0_C1)
  Cast To Single57/1 -> SignalBusCreator/104(L1_C2)
  Ground53/1 -> Cast To Single113/1
  LLClb/1(LLClb_bsLLClb) -> [bsLLClb]
  Ground23/1 -> Cast To Single32/1
  Cast To Single102/1 -> SignalBusCreator/74(O_R1_LC)
  Ground62/1 -> Cast To Single116/1
  Ground43/1 -> Cast To Single39/1
  Ground69/1 -> Cast To Single62/1
  LKASve_g_IMAP_L0_C0/1 -> Cast To Single41/1
  Cast To Single15/1 -> SignalBusCreator/38(O_L0_C0)
  Ground13/1 -> Cast To Single10/1
  LKASve_d_IMAP_TCU_ActualGear/1 -> Cast To Single84/1
  Cast To Single79/1 -> SignalBusCreator/15(ESC_YawRate_Valid)
  Cast To Single95/1 -> SignalBusCreator/50(O_L1_Type)
  Cast To Single99/1 -> SignalBusCreator/64(O_R0_LC)
  Cast To Single13/1 -> SignalBusCreator/36(O_L0_C2)
  LKASve_g_IMAP_SW_Angle_Speed/1 -> Cast To Single9/1
  Ground33/1 -> Cast To Single26/1
  Ground63/1 -> Cast To Single117/1
  Cast To Single45/1 -> SignalBusCreator/84(L0_VR)
  Cast To Single98/1 -> SignalBusCreator/60(O_R0_Type)
  [bsInInfo] -> LL/1(bsInInfo)
  Cast To Single113/1 -> SignalBusCreator/98(R0_C)
  Cast To Single91/1 -> SignalBusCreator/39(O_L0_Q)
  Ground24/1 -> Cast To Single31/1
  Cast To Single54/1 -> SignalBusCreator/100(R0_TLC)
  Ground48/1 -> Cast To Single106/1
  LKASve_g_IMAP_O_R0_VR/1 -> Cast To Single24/1
  LKASve_g_IMAP_O_L0_C3/1 -> Cast To Single12/1
  EPS_State_Mashine/1(EPS_Ctr_State) -> Memory/1
  Cast To Single116/1 -> SignalBusCreator/108(L1_Type)
  Cast To Single123/1 -> SignalBusCreator/124(CameraSynFault)
  LKASve_g_IMAP_SW_Angle/1 -> Cast To Single8/1
  Cast To Single124/1 -> SignalBusCreator/125(Camera_Status)
  Memory/1 -> [EPS_LKA_State]
  Cast To Single26/1 -> SignalBusCreator/63(O_R0_W)
  Cast To Single117/1 -> SignalBusCreator/109(L1_C)
  Cast To Single/1 -> SignalBusCreator/5(EPS_SW_Trq)
  Cast To Single104/1 -> SignalBusCreator/76(Fusion_Status)
  Ground20/1 -> Cast To Single90/1
  Ground35/1 -> Cast To Single33/1
  Cast To Single111/1 -> SignalBusCreator/96(R0_Q)
  Ground60/1 -> Cast To Single59/1
  Cast To Single28/1 -> SignalBusCreator/51(O_L1_VR)
  Ground7/1 -> Cast To Single78/1
  Cast To Single32/1 -> SignalBusCreator/45(O_L1_C3)
  Ground6/1 -> Cast To Single1/1
  Cast To Single109/1 -> SignalBusCreator/87(L0_C)
  Ground42/1 -> Cast To Single38/1
  LKASve_g_IMAP_O_L0_VR/1 -> Cast To Single16/1
  Cast To Single62/1 -> SignalBusCreator/115(R1_C2)
  Cast To Single64/1 -> SignalBusCreator/117(R1_VR)
  LKASve_d_IMAP_BCM_Double_Light/1 -> Cast To Single81/1
  LKASve_g_IMAP_R0_C2/1 -> Cast To Single50/1
  Cast To Single59/1 -> SignalBusCreator/106(L1_VR)
  Cast To Single37/1 -> SignalBusCreator/71(O_R1_VR)
  Cast To Single92/1 -> SignalBusCreator/40(O_L0_Type)
  LKASve_g_IMAP_L0_VR/1 -> Cast To Single45/1
  Ground5/1 -> Cast To Single76/1
  Ground51/1 -> Cast To Single46/1
  Ground32/1 -> Cast To Single96/1
  LKASve_d_IMAP_L0_Q/1 -> Cast To Single107/1
  Cast To Single122/1 -> SignalBusCreator/123(R1_LC)
  LKASve_g_IMAP_R0_C3/1 -> Cast To Single51/1
  Cast To Single58/1 -> SignalBusCreator/105(L1_C3)
  Cast To Single20/1 -> SignalBusCreator/55(O_R0_C3)
  Cast To Single118/1 -> SignalBusCreator/112(L1_LC)
  Cast To Single6/1 -> SignalBusCreator/18(ESC_LonAcc)
  LKASve_d_IMAP_R0_Type/1 -> Cast To Single112/1
  LKASve_g_IMAP_ESC_YawRate/1 -> Cast To Single3/1
  Cast To Single86/1 -> SignalBusCreator/29(SAS_In_Status)
  Ground1/1 -> Cast To Single72/1
  Cast To Single30/1 -> SignalBusCreator/47(O_L1_C1)
  Cast To Single94/1 -> SignalBusCreator/49(O_L1_Q)
  Cast To Single63/1 -> SignalBusCreator/116(R1_C3)
  Cast To Single8/1 -> SignalBusCreator/21(SW_Angle)
  Cast To Single47/1 -> SignalBusCreator/89(L0_TLC)
  Cast To Single69/1 -> SignalBusCreator/2(LKA_Mode)
  LKASve_d_IMAP_Camera_Status/1 -> Cast To Single124/1
  Cast To Single29/1 -> SignalBusCreator/48(O_L1_C0)
  LKASve_d_IMAP_EPS_LKA_State/1 -> ?
  ADAS_541_PSA1__LDW_Flag/1 -> ?
  ADAS_541_PSA1__Vehicle_Lane_Display/1 -> ?
  ADAS_3F2_PSA1__Column_angle_setpoint3F2/1 -> ?
  LKASve_g_IMAP_L0_C3/1 -> Cast To Single44/1
  Ground38/1 -> Cast To Single36/1
  Cast To Single53/1 -> SignalBusCreator/99(R0_W)
  Ground52/1 -> Cast To Single110/1
  Cast To Single97/1 -> SignalBusCreator/59(O_R0_Q)
  LKASve_g_IMAP_O_L0_C0/1 -> Cast To Single15/1
  LKASve_g_IMAP_O_R0_C2/1 -> Cast To Single21/1
  LKASve_g_IMAP_ESC_Brake_Press/1 -> Cast To Single7/1
  Cast To Single101/1 -> SignalBusCreator/70(O_R1_Type)
  Cast To Single48/1 -> SignalBusCreator/91(R0_C0)
  LKASve_g_IMAP_ESC_VehSpd/1 -> Cast To Single5/1
  Cast To Single67/1 -> SignalBusCreator/121(R1_W)
  Ground39/1 -> Cast To Single100/1
  Cast To Single93/1 -> SignalBusCreator/44(O_L0_LC)
  Ground21/1 -> Cast To Single18/1
  Cast To Single83/1 -> SignalBusCreator/25(BCM_Right_Light)
  Cast To Single74/1 -> SignalBusCreator/8(SAS_Clb_State)
  Cast To Single121/1 -> SignalBusCreator/120(R1_C)
  Ground71/1 -> Cast To Single64/1
  Cast To Single36/1 -> SignalBusCreator/68(O_R1_C0)
  Cast To Single40/1 -> SignalBusCreator/79(ConsArea)
  Cast To Single12/1 -> SignalBusCreator/35(O_L0_C3)
  SignalBusCreator/1(bsInInfo) -> [bsInInfo]
  Ground30/1 -> Cast To Single27/1
  Ground16/1 -> Cast To Single87/1
  Ground8/1 -> Cast To Single79/1
  Cast To Single50/1 -> SignalBusCreator/93(R0_C2)
  Ground74/1 -> Cast To Single121/1
  Ground3/1 -> Cast To Single74/1
  Cast To Single1/1 -> SignalBusCreator/11(EPS_LKA_Current)
  LKASve_d_IMAP_O_R0_Type/1 -> Cast To Single98/1
  Cast To Single7/1 -> SignalBusCreator/20(ESC_Brake_Press)
  Ground12/1 -> Cast To Single83/1
  LKASve_g_IMAP_L0_C2/1 -> Cast To Single43/1
  Cast To Single105/1 -> SignalBusCreator/77(Lane_Valid)
  Ground18/1 -> Cast To Single89/1
  [EPS_LKA_State] -> Cast To Single77/1
  LKASve_g_IMAP_L0_TLC/1 -> Cast To Single47/1
  LKASve_g_IMAP_O_L0_C2/1 -> Cast To Single13/1
  Cast To Single71/1 -> SignalBusCreator/3(LDW_Warn_Mode)
  Cast To Single66/1 -> SignalBusCreator/111(L1_TLC)
  Ground66/1 -> Cast To Single118/1
  LKASve_g_IMAP_ESC_LonAcc/1 -> Cast To Single6/1
  LKASve_d_IMAP_O_R0_Q/1 -> Cast To Single97/1
  Ground64/1 -> Cast To Single65/1
  Ground37/1 -> Cast To Single35/1
  Cast To Single55/1 -> SignalBusCreator/102(L1_C0)
  Cast To Single120/1 -> SignalBusCreator/119(R1_Type)
  Cast To Single112/1 -> SignalBusCreator/97(R0_Type)
  Cast To Single115/1 -> SignalBusCreator/107(L1_Q)
  Cast To Single110/1 -> SignalBusCreator/90(L0_LC)
  ADAS_3F2_PSA1__Permit_to_know_if_LKA_or_LPA3F2/1 -> ?
  Cast To Single27/1 -> SignalBusCreator/52(O_L1_TLC)
  Cast To Single119/1 -> SignalBusCreator/118(R1_Q)
  Ground/1 -> Cast To Single71/1
  Cast To Single44/1 -> SignalBusCreator/83(L0_C3)
  Ground14/1 -> Cast To Single85/1
  LKASve_g_IMAP_R0_C1/1 -> Cast To Single49/1
  Cast To Single87/1 -> SignalBusCreator/30(ESC_VehSpd_Valid)
  Cast To Single75/1 -> SignalBusCreator/9(SAS_Trim_State)
  Cast To Single89/1 -> SignalBusCreator/32(O_Lane_Valid)
  Ground40/1 -> Cast To Single101/1
  LKASve_d_IMAP_R0_Q/1 -> Cast To Single111/1
  Cast To Single76/1 -> SignalBusCreator/10(EPS_TrqLim_State)
  LKASve_g_IMAP_O_R0_TLC/1 -> Cast To Single25/1
  Ground72/1 -> Cast To Single119/1
  Ground47/1 -> Cast To Single105/1
  Cast To Single108/1 -> SignalBusCreator/86(L0_Type)
  Cast To Single14/1 -> SignalBusCreator/37(O_L0_C1)
  Cast To Single100/1 -> SignalBusCreator/69(O_R1_Q)
  Cast To Single10/1 -> SignalBusCreator/26(AccPedal_Pos)
  Ground2/1 -> Cast To Single73/1
  Cast To Single33/1 -> SignalBusCreator/65(O_R1_C3)
  Cast To Single38/1 -> SignalBusCreator/72(O_R1_TLC)
  Cast To Single41/1 -> SignalBusCreator/80(L0_C0)
  Cast To Single17/1 -> SignalBusCreator/42(O_L0_TLC)
  Cast To Single84/1 -> SignalBusCreator/27(TCU_ActualGear)
  Ground36/1 -> Cast To Single34/1
  Ground41/1 -> Cast To Single37/1
  Ground49/1 -> Cast To Single40/1
  Ground11/1 -> Cast To Single82/1
  Ground59/1 -> Cast To Single58/1
  Cast To Single21/1 -> SignalBusCreator/56(O_R0_C2)
  Ground9/1 -> Cast To Single4/1
  Cast To Single65/1 -> SignalBusCreator/110(L1_W)
  Cast To Single56/1 -> SignalBusCreator/103(L1_C1)
  Cast To Single72/1 -> SignalBusCreator/6(EPS_Error_State)
  Ground4/1 -> Cast To Single75/1
  Ground65/1 -> Cast To Single66/1
  Cast To Single11/1 -> SignalBusCreator/33(O_Lane_ConsArea)
  LKASve_g_IMAP_O_R0_C0/1 -> Cast To Single23/1
  LKASve_g_IMAP_R0_TLC/1 -> Cast To Single54/1
  Cast To Single46/1 -> SignalBusCreator/88(L0_W)
  Cast To Single19/1 -> SignalBusCreator/53(O_L1_W)
  LKASve_d_IMAP_L0_Type/1 -> Cast To Single108/1
  Cast To Single103/1 -> SignalBusCreator/75(Sensor_Status)
  LKASve_g_IMAP_EPS_SW_Trq/1 -> Cast To Single/1
  Cast To Single5/1 -> SignalBusCreator/17(ESC_VehSpd)
  Ground29/1 -> Cast To Single28/1
  LKASve_g_IMAP_ESC_LatAcc/1 -> Cast To Single2/1
  Cast To Single52/1 -> SignalBusCreator/95(R0_VR)
  LKASve_g_IMAP_R0_VR/1 -> Cast To Single52/1
  Ground55/1 -> Cast To Single114/1
  Cast To Single25/1 -> SignalBusCreator/62(O_R0_TLC)
  Ground50/1 -> Cast To Single109/1
  Cast To Single39/1 -> SignalBusCreator/73(O_R1_W)
  Cast To Single96/1 -> SignalBusCreator/54(O_L1_LC)
  Ground57/1 -> Cast To Single56/1
  Ground54/1 -> Cast To Single53/1
  Ground17/1 -> Cast To Single88/1
  Ground46/1 -> Cast To Single104/1
  Ground73/1 -> Cast To Single120/1
  Ground78/1 -> Cast To Single123/1
  Ground45/1 -> Cast To Single103/1
  Cast To Single2/1 -> SignalBusCreator/12(ESC_LatAcc)
  Ground77/1 -> Cast To Single122/1
  [bsLLOut] -> Output/1(bsLLOut)
  Ground25/1 -> Cast To Single30/1
  LKASve_d_IMAP_LKA_Main_Switch/1 -> Cast To Single70/1
  Ground28/1 -> Cast To Single95/1
  Cast To Single90/1 -> SignalBusCreator/34(O_Lane_RoadType)
  LKASve_g_IMAP_L0_C1/1 -> Cast To Single42/1
  Cast To Single42/1 -> SignalBusCreator/81(L0_C1)
  Ground58/1 -> Cast To Single57/1
  Ground68/1 -> Cast To Single61/1
  Ground44/1 -> Cast To Single102/1
  Cast To Single31/1 -> SignalBusCreator/46(O_L1_C2)
  Cast To Single114/1 -> SignalBusCreator/101(R0_LC)
  Cast To Single85/1 -> SignalBusCreator/28(SWS_Fault_Code)
  LKASve_d_IMAP_LKA_Mode/1 -> Cast To Single69/1
  Cast To Single82/1 -> SignalBusCreator/24(BCM_Left_Light)
  Ground67/1 -> Cast To Single60/1
  Cast To Single9/1 -> SignalBusCreator/22(SW_Angle_Speed)
  Ground27/1 -> Cast To Single94/1
  Cast To Single23/1 -> SignalBusCreator/58(O_R0_C0)
  Cast To Single70/1 -> SignalBusCreator/1(LKA_Main_Switch)
  Cast To Single88/1 -> SignalBusCreator/31(EPS_SWHold_State)
  Ground15/1 -> Cast To Single86/1
  Ground19/1 -> Cast To Single11/1
  Cast To Single61/1 -> SignalBusCreator/114(R1_C1)
  Cast To Single81/1 -> SignalBusCreator/23(BCM_Double_Light)
  Cast To Single106/1 -> SignalBusCreator/78(Road_Type)
  LKASve_g_IMAP_O_R0_C3/1 -> Cast To Single20/1
  [bsLLClb] -> LL/2(bsLLClb)
  Cast To Single78/1 -> SignalBusCreator/13(ESC_LatAcc_Valid)
  Cast To Single3/1 -> SignalBusCreator/14(ESC_YawRate)
  Ground26/1 -> Cast To Single29/1
  LL/1(bsLLOut) -> [bsLLOut]
  Cast To Single68/1 -> SignalBusCreator/122(R1_TLC)
  Cast To Single51/1 -> SignalBusCreator/94(R0_C3)
  Ground22/1 -> Cast To Single93/1
  Cast To Single24/1 -> SignalBusCreator/61(O_R0_VR)
  Ground76/1 -> Cast To Single68/1
  LKASve_d_IMAP_O_L0_Q/1 -> Cast To Single91/1
  Cast To Single18/1 -> SignalBusCreator/43(O_L0_W)
  Ground34/1 -> Cast To Single99/1
  LKASve_g_IMAP_R0_C0/1 -> Cast To Single48/1
  LKASve_g_IMAP_O_R0_C1/1 -> Cast To Single22/1
  Ground56/1 -> Cast To Single55/1
  Cast To Single35/1 -> SignalBusCreator/67(O_R1_C1)
  Cast To Single43/1 -> SignalBusCreator/82(L0_C2)
  Ground10/1 -> Cast To Single80/1
  Output/1(Vehicle_Lane_Display) -> LKASve_y_Vehicle_Lane_Display/1  "LKASve_y_Vehicle_Lane_Display"
  Output/2(LDW_Status_Display) -> LKASve_y_LDW_Status_Display/1  "LKASve_y_LDW_Status_Display"
  Output/3(LKA_Status_Display) -> LKASve_y_LKA_Status_Display/1  "LKASve_y_LKA_Status_Display"
  Output/4(LDW_Flag) -> LKASve_y_LDW_Flag/1  "LKASve_y_LDW_Flag"
  Output/5(Hands_Off_Warning) -> LKASve_y_Hands_Off_Warning/1  "LKASve_y_Hands_Off_Warning"
  Output/6(LKA_Action_Indication) -> LKASve_y_LKA_Action_Indication/1  "LKASve_y_LKA_Action_Indication"
  Output/7(HMI_Popup_Status) -> LKASve_y_HMI_Popup_Status/1  "LKASve_y_HMI_Popup_Status"
  Output/8(EPS_State_Control) -> LKAve_y_EPS_State_Control/1, EPS_State_Mashine/1(LKA_State2EPS)  "LKASve_y_EPS_State_Control"
  Output/9(LKA_SWA_Control) -> LKASve_g_LKA_SWA_Control/1  "LKASve_g_LKA_SWA_Control"
  Output/10(EPS_Factor_Control) -> LKASve_g_EPS_Factor_Control/1  "LKASve_g_EPS_Factor_Control"
  Output/11(EPS_LKA_Control) -> LKASve_y_EPS_LKA_Control/1  "LKASve_y_EPS_LKA_Control"

== system LKAS_SIL/EPS_State_Mashine ==
  LKA_State2EPS : Inport
  Data Type Conversion2 : DataTypeConversion  OutDataTypeStr=uint16
  Steering Angle Cmd Synthesis State Machine (SWASynSM) : Stateflow chart  TreatAsAtomicUnit=on
  EPS_Ctr_State : Outport
  wires:
  LKA_State2EPS/1 -> Data Type Conversion2/1
  Steering Angle Cmd Synthesis State Machine (SWASynSM)/1(EPS_Ctr_State) -> EPS_Ctr_State/1
  Data Type Conversion2/1 -> Steering Angle Cmd Synthesis State Machine (SWASynSM)/1(LKA_State2EPS)

== system LKAS_SIL/LL ==
  bsInInfo : Inport
  bsLLClb : Inport  Port=2
  Bus Selector1 : BusSelector  OutputSignals=bsLaneInfo.bsR0Info.R0_Q,bsLaneInfo.bsL0Info.L0_Q
  Bus Selector2 : BusSelector  OutputSignals=bsEPSInfo
  Bus Selector3 : BusSelector  OutputSignals=LKA_State,LDW_State
  Bus Selector4 : BusSelector  OutputSignals=bsLaneInfo.Fusion_AdditionalInf.Carema_Status
  Fault_Diagnostic : Subsystem
  Ground1 : Ground
  Ground3 : Ground
  Human Machine Interface (HMI) : Subsystem
  LL Inputs Mapping : Subsystem
  LL Output (LLOut) : Subsystem
  LLOn : Subsystem
  Subsystem : Subsystem
  Terminator : Terminator
  Version : Constant  Value=200918  OutMin=20410  OutMax=220630  OutDataTypeStr=single
  bsLLOut : Outport
  tag scope: LLMon=global
  wires:
  LLOn/5(LLMon) -> [LLMon]
  [bsInInfo] -> Fault_Diagnostic/1(bsInInfo)
  Fault_Diagnostic/1(bsSignalFault) -> [bsSignalFault]
  LLOn/4(M) -> [LLOn_M]
  [bsInfo] -> LLOn/2(bsInInfo)
  [bsSignalFault] -> LLOn/4(bsSignalFault)
  LLOn/3(phiSWACmd) -> [LLOn_phiSWACmd]
  LLOn/1(bsLLState) -> [LLOn_bsLLState]
  [bsLLClb] -> LLOn/3(bsLLClb)
  Subsystem/2(Mode) -> [LLOn_stDACMode], LLOn/1(stDACMode)
  [HMI_bsLLHMI] -> LL Output (LLOut)/3(LLOut_bsLLHMI)
  [LLOn_phiSWACmd] -> LL Output (LLOut)/2(LLOut_phiSWACmd)
  [bsInfo] -> Bus Selector1/1, Bus Selector2/1, Bus Selector4/1
  [bsInfo] -> Subsystem/1(bsInfo)
  Ground1/1 -> Human Machine Interface (HMI)/8(HMI_camera_common_fault)
  Bus Selector4/1 -> Human Machine Interface (HMI)/9(HMI_Front_Camera_Blocked)  "<Carema_Status>"
  [LLOn_M] -> LL Output (LLOut)/4(LLOut_M)
  Bus Selector3/2 -> Human Machine Interface (HMI)/4(HMI_LDW_STATE)  "<LDW_State>"
  bsLLClb/1 -> [bsLLClb]
  [LLOn_bsLLState] -> LL Output (LLOut)/1(LLOut_bsLLState)
  Bus Selector1/1 -> Human Machine Interface (HMI)/5(HMI_R0_Quality)  "<R0_Q>"
  LLOn/2(LDW_Flag) -> [LLOn_bsLDWWarnInfo]
  Bus Selector3/1 -> Human Machine Interface (HMI)/3(HMI_LKA_STATE)  "<LKA_State>"
  Bus Selector1/2 -> Human Machine Interface (HMI)/6(HMI_L0_Quality)  "<L0_Q>"
  [LLOn_stDACMode] -> Human Machine Interface (HMI)/1(HMI_stDACmode)
  LL Inputs Mapping/1(bsInfo) -> [bsInfo]
  [bsInInfo] -> LL Inputs Mapping/1(bsInInfo)
  [LLOn_bsLLState] -> Bus Selector3/1
  Version/1 -> Terminator/1  "ob_LKA_Version"
  LL Output (LLOut)/1(LL_bsLLOut) -> bsLLOut/1  "bsLLOut"
  Subsystem/1(On) -> LLOn/Enable
  Bus Selector2/1 -> Human Machine Interface (HMI)/7(HMI_EPSInfo)  "<bsEPSInfo>"
  [LLOn_bsLDWWarnInfo] -> Human Machine Interface (HMI)/2(HMI_LDWWarn)
  Human Machine Interface (HMI)/1(HMI_LDWLKA) -> [HMI_bsLLHMI]  "bsLLHMI"
  Ground3/1 -> Human Machine Interface (HMI)/10(HMI_stFaultCSyn)
  bsInInfo/1 -> [bsInInfo]

== system LKAS_SIL/LLClb ==
  Bus Creator : BusCreator  Inputs=4
  ConstantClb : Subsystem
  LDWClb : Subsystem
  LKAClb : Subsystem
  LLSMConClb : Subsystem
  LLClb_bsLLClb : Outport
  wires:
  LKAClb/1(LKAClb) -> Bus Creator/3  "bsLKAClb"
  LDWClb/1(LDWClb) -> Bus Creator/2  "bsLDWClb"
  Bus Creator/1 -> LLClb_bsLLClb/1  "bsLLClb"
  LLSMConClb/1(LLSMConClb) -> Bus Creator/1  "bsLLSMConClb"
  ConstantClb/1(ConstantClb) -> Bus Creator/4  "bsConstantClb"

== system LKAS_SIL/Output ==
  bsLLOut : Inport
  Bus Selector : BusSelector  OutputSignals=Vehicle_Lane_Display,LDW_Status_Display,LKA_Status_Display,LDW_Flag,Hands_off_warning,LKA_action_indication,HMI_Popup_Status,EPS_State_Ctl,LMS_phiSWACmd,Coefficient_toregulate_EPS,Permit_to_know_if_LKA_or_LPA3F2
  Vehicle_Lane_Display : Outport
  LDW_Status_Display : Outport  Port=2
  LKA_Status_Display : Outport  Port=3
  LDW_Flag : Outport  Port=4
  Hands_Off_Warning : Outport  Port=5
  LKA_Action_Indication : Outport  Port=6
  HMI_Popup_Status : Outport  Port=7
  EPS_State_Control : Outport  Port=8
  LKA_SWA_Control : Outport  Port=9
  EPS_Factor_Control : Outport  Port=10
  EPS_LKA_Control : Outport  Port=11
  wires:
  bsLLOut/1 -> Bus Selector/1
  Bus Selector/1 -> Vehicle_Lane_Display/1  "<Vehicle_Lane_Display>"
  Bus Selector/2 -> LDW_Status_Display/1  "<LDW_Status_Display>"
  Bus Selector/3 -> LKA_Status_Display/1  "<LKA_Status_Display>"
  Bus Selector/4 -> LDW_Flag/1  "<LDW_Flag>"
  Bus Selector/5 -> Hands_Off_Warning/1  "<Hands_off_warning>"
  Bus Selector/6 -> LKA_Action_Indication/1  "<LKA_action_indication>"
  Bus Selector/7 -> HMI_Popup_Status/1  "<HMI_Popup_Status>"
  Bus Selector/8 -> EPS_State_Control/1  "<EPS_State_Ctl>"
  Bus Selector/9 -> LKA_SWA_Control/1  "<LMS_phiSWACmd>"
  Bus Selector/10 -> EPS_Factor_Control/1  "<Coefficient_toregulate_EPS>"
  Bus Selector/11 -> EPS_LKA_Control/1  "<Permit_to_know_if_LKA_or_LPA3F2>"

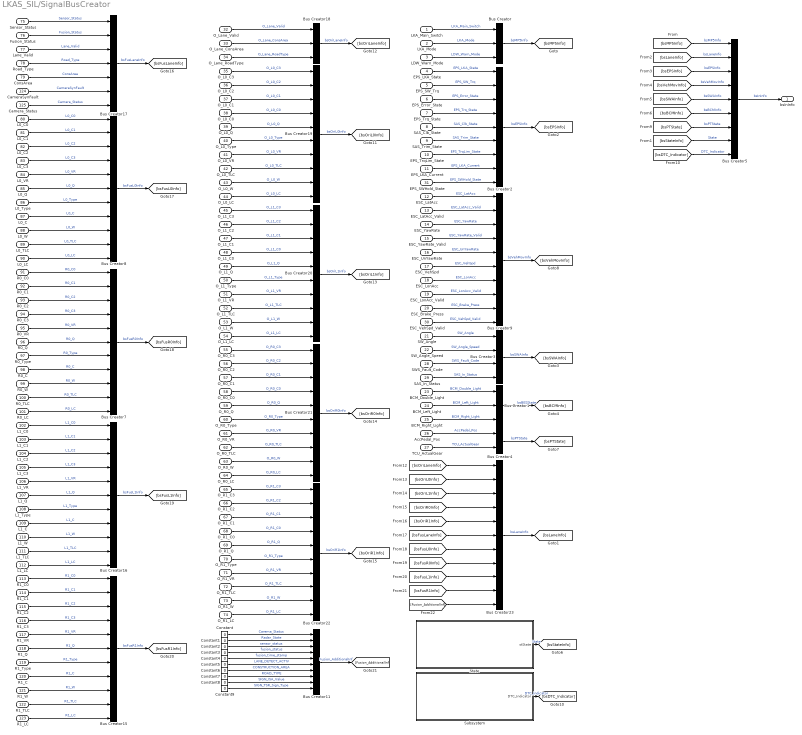
== system LKAS_SIL/SignalBusCreator ==
  LKA_Main_Switch : Inport
  LKA_Mode : Inport  Port=2
  LDW_Warn_Mode : Inport  Port=3
  EPS_LKA_State : Inport  Port=4
  EPS_SW_Trq : Inport  Port=5
  EPS_Error_State : Inport  Port=6
  EPS_Trq_State : Inport  Port=7
  SAS_Clb_State : Inport  Port=8
  SAS_Trim_State : Inport  Port=9
  EPS_TrqLim_State : Inport  Port=10
  EPS_LKA_Current : Inport  Port=11
  ESC_LatAcc : Inport  Port=12
  ESC_LatAcc_Valid : Inport  Port=13
  ESC_YawRate : Inport  Port=14
  ESC_YawRate_Valid : Inport  Port=15
  ESC_UnYawRate : Inport  Port=16
  ESC_VehSpd : Inport  Port=17
  ESC_LonAcc : Inport  Port=18
  ESC_LonAcc_Valid : Inport  Port=19
  ESC_Brake_Press : Inport  Port=20
  SW_Angle : Inport  Port=21
  SW_Angle_Speed : Inport  Port=22
  BCM_Double_Light : Inport  Port=23
  BCM_Left_Light : Inport  Port=24
  BCM_Right_Light : Inport  Port=25
  AccPedal_Pos : Inport  Port=26
  TCU_ActualGear : Inport  Port=27
  SWS_Fault_Code : Inport  Port=28
  SAS_In_Status : Inport  Port=29
  ESC_VehSpd_Valid : Inport  Port=30
  EPS_SWHold_State : Inport  Port=31
  O_Lane_Valid : Inport  Port=32
  O_Lane_ConsArea : Inport  Port=33
  O_Lane_RoadType : Inport  Port=34
  O_L0_C3 : Inport  Port=35
  O_L0_C2 : Inport  Port=36
  O_L0_C1 : Inport  Port=37
  O_L0_C0 : Inport  Port=38
  O_L0_Q : Inport  Port=39
  O_L0_Type : Inport  Port=40
  O_L0_VR : Inport  Port=41
  O_L0_TLC : Inport  Port=42
  O_L0_W : Inport  Port=43
  O_L0_LC : Inport  Port=44
  O_L1_C3 : Inport  Port=45
  O_L1_C2 : Inport  Port=46
  O_L1_C1 : Inport  Port=47
  O_L1_C0 : Inport  Port=48
  O_L1_Q : Inport  Port=49
  O_L1_Type : Inport  Port=50
  O_L1_VR : Inport  Port=51
  O_L1_TLC : Inport  Port=52
  O_L1_W : Inport  Port=53
  O_L1_LC : Inport  Port=54
  O_R0_C3 : Inport  Port=55
  O_R0_C2 : Inport  Port=56
  O_R0_C1 : Inport  Port=57
  O_R0_C0 : Inport  Port=58
  O_R0_Q : Inport  Port=59
  O_R0_Type : Inport  Port=60
  O_R0_VR : Inport  Port=61
  O_R0_TLC : Inport  Port=62
  O_R0_W : Inport  Port=63
  O_R0_LC : Inport  Port=64
  O_R1_C3 : Inport  Port=65
  O_R1_C2 : Inport  Port=66
  O_R1_C1 : Inport  Port=67
  O_R1_C0 : Inport  Port=68
  O_R1_Q : Inport  Port=69
  O_R1_Type : Inport  Port=70
  O_R1_VR : Inport  Port=71
  O_R1_TLC : Inport  Port=72
  O_R1_W : Inport  Port=73
  O_R1_LC : Inport  Port=74
  Sensor_Status : Inport  Port=75
  Fusion_Status : Inport  Port=76
  Lane_Valid : Inport  Port=77
  Road_Type : Inport  Port=78
  ConsArea : Inport  Port=79
  L0_C0 : Inport  Port=80
  L0_C1 : Inport  Port=81
  L0_C2 : Inport  Port=82
  L0_C3 : Inport  Port=83
  L0_VR : Inport  Port=84
  L0_Q : Inport  Port=85
  L0_Type : Inport  Port=86
  L0_C : Inport  Port=87
  L0_W : Inport  Port=88
  L0_TLC : Inport  Port=89
  L0_LC : Inport  Port=90
  R0_C0 : Inport  Port=91
  R0_C1 : Inport  Port=92
  R0_C2 : Inport  Port=93
  R0_C3 : Inport  Port=94
  R0_VR : Inport  Port=95
  R0_Q : Inport  Port=96
  R0_Type : Inport  Port=97
  R0_C : Inport  Port=98
  R0_W : Inport  Port=99
  R0_TLC : Inport  Port=100
  R0_LC : Inport  Port=101
  L1_C0 : Inport  Port=102
  L1_C1 : Inport  Port=103
  L1_C2 : Inport  Port=104
  L1_C3 : Inport  Port=105
  L1_VR : Inport  Port=106
  L1_Q : Inport  Port=107
  L1_Type : Inport  Port=108
  L1_C : Inport  Port=109
  L1_W : Inport  Port=110
  L1_TLC : Inport  Port=111
  L1_LC : Inport  Port=112
  R1_C0 : Inport  Port=113
  R1_C1 : Inport  Port=114
  R1_C2 : Inport  Port=115
  R1_C3 : Inport  Port=116
  R1_VR : Inport  Port=117
  R1_Q : Inport  Port=118
  R1_Type : Inport  Port=119
  R1_C : Inport  Port=120
  R1_W : Inport  Port=121
  R1_TLC : Inport  Port=122
  R1_LC : Inport  Port=123
  CameraSynFault : Inport  Port=124
  Camera_Status : Inport  Port=125
  Bus Creator : BusCreator  Inputs=3
  Bus Creator1 : BusCreator  Inputs=3
  Bus Creator{9,11,19..22} (6 alike) : BusCreator  Inputs=10
  Bus Creator{7..8,15..16,23} (5 alike) : BusCreator  Inputs=11
  Bus Creator17 : BusCreator  Inputs=7
  Bus Creator18 : BusCreator  Inputs=3
  Bus Creator2 : BusCreator  Inputs=9
  Bus Creator3 : BusCreator  Inputs=4
  Bus Creator4 : BusCreator  Inputs=2
  Bus Creator5 : BusCreator  Inputs=9
  Constant{,1..9} (10 alike) : Constant  Value=0  OutDataTypeStr=uint8
  State : Subsystem
  Subsystem : Subsystem
  bsInInfo : Outport
  wires:
  Bus Creator9/1 -> [bsVehMovInfo]  "bsVehMovInfo"
  Bus Creator3/1 -> [bsSWAInfo]  "bsSWAInfo"
  Bus Creator1/1 -> [bsBCMInfo]  "bsBESState"
  Bus Creator2/1 -> [bsEPSInfo]  "bsEPSInfo"
  Bus Creator/1 -> [bsMP5Info]  "bsMP5Info"
  [bsLaneInfo] -> Bus Creator5/2  "bsLaneInfo"
  [bsEPSInfo] -> Bus Creator5/3  "bsEPSInfo"
  [bsVehMovInfo] -> Bus Creator5/4  "bsVehMovInfo"
  [bsSWAInfo] -> Bus Creator5/5  "bsSWAInfo"
  [bsBCMInfo] -> Bus Creator5/6  "bsBCMInfo"
  [bsPTState] -> Bus Creator5/7  "bsPTState"
  ESC_Brake_Press/1 -> Bus Creator9/9  "ESC_Brake_Press"
  ESC_LatAcc/1 -> Bus Creator9/1  "ESC_LatAcc"
  ESC_YawRate/1 -> Bus Creator9/3  "ESC_YawRate"
  ESC_VehSpd/1 -> Bus Creator9/6  "ESC_VehSpd"
  ESC_LonAcc/1 -> Bus Creator9/7  "ESC_LonAcc"
  EPS_SW_Trq/1 -> Bus Creator2/2  "EPS_SW_Trq"
  LKA_Main_Switch/1 -> Bus Creator/1  "LKA_Main_Switch"
  LKA_Mode/1 -> Bus Creator/2  "LKA_Mode"
  SW_Angle/1 -> Bus Creator3/1  "SW_Angle"
  SW_Angle_Speed/1 -> Bus Creator3/2  "SW_Angle_Speed"
  [bsMP5Info] -> Bus Creator5/1  "bsMP5Info"
  [bsStateInfo] -> Bus Creator5/8  "State"
  [bsDTC_Indicator] -> Bus Creator5/9  "DTC_Indicator"
  L0_C1/1 -> Bus Creator8/2  "L0_C1"
  L0_TLC/1 -> Bus Creator8/10  "L0_TLC"
  L0_C0/1 -> Bus Creator8/1  "L0_C0"
  L0_Q/1 -> Bus Creator8/6  "L0_Q"
  L0_C2/1 -> Bus Creator8/3  "L0_C2"
  L0_W/1 -> Bus Creator8/9  "L0_W"
  L0_C3/1 -> Bus Creator8/4  "L0_C3"
  L0_VR/1 -> Bus Creator8/5  "L0_VR"
  L0_LC/1 -> Bus Creator8/11  "L0_LC"
  Constant6/1 -> Bus Creator11/7  "CONSTRUCTION_AREA"
  Constant4/1 -> Bus Creator11/5  "fusion_time_stamp"
  L0_Type/1 -> Bus Creator8/7  "L0_Type"
  Constant5/1 -> Bus Creator11/6  "LANE_DETECT_ACTIV"
  Constant1/1 -> Bus Creator11/2  "Radar_State"
  Constant7/1 -> Bus Creator11/8  "ROAD_TYPE"
  Constant8/1 -> Bus Creator11/9  "SIGN_ISA_Value"
  Constant3/1 -> Bus Creator11/4  "fusion_status"
  Constant2/1 -> Bus Creator11/3  "sensor_status"
  Constant/1 -> Bus Creator11/1  "Carema_Status"
  Constant9/1 -> Bus Creator11/10  "SIGN_TSR_Sign_Type"
  LDW_Warn_Mode/1 -> Bus Creator/3  "LDW_Warn_Mode"
  EPS_LKA_State/1 -> Bus Creator2/1  "EPS_LKA_State"
  EPS_Error_State/1 -> Bus Creator2/3  "EPS_Error_State"
  EPS_Trq_State/1 -> Bus Creator2/4  "EPS_Trq_State"
  SAS_Clb_State/1 -> Bus Creator2/5  "SAS_Clb_State"
  SAS_Trim_State/1 -> Bus Creator2/6  "SAS_Trim_State"
  EPS_TrqLim_State/1 -> Bus Creator2/7  "EPS_TrqLim_State"
  EPS_LKA_Current/1 -> Bus Creator2/8  "EPS_LKA_Current"
  ESC_LatAcc_Valid/1 -> Bus Creator9/2  "ESC_LatAcc_Valid"
  ESC_YawRate_Valid/1 -> Bus Creator9/4  "ESC_YawRate_Valid"
  ESC_UnYawRate/1 -> Bus Creator9/5  "ESC_UnYawRate"
  ESC_LonAcc_Valid/1 -> Bus Creator9/8  "ESC_LonAcc_Valid"
  BCM_Double_Light/1 -> Bus Creator1/1  "BCM_Double_Light"
  BCM_Left_Light/1 -> Bus Creator1/2  "BCM_Left_Light"
  BCM_Right_Light/1 -> Bus Creator1/3  "BCM_Right_Light"
  Bus Creator4/1 -> [bsPTState]  "bsPTState"
  AccPedal_Pos/1 -> Bus Creator4/1  "AccPedal_Pos"
  TCU_ActualGear/1 -> Bus Creator4/2  "TCU_ActualGear"
  SWS_Fault_Code/1 -> Bus Creator3/3  "SWS_Fault_Code"
  SAS_In_Status/1 -> Bus Creator3/4  "SAS_In_Status"
  ESC_VehSpd_Valid/1 -> Bus Creator9/10  "ESC_VehSpd_Valid"
  EPS_SWHold_State/1 -> Bus Creator2/9  "EPS_SWHold_State"
  L0_C/1 -> Bus Creator8/8  "L0_C"
  R0_C/1 -> Bus Creator7/8  "R0_C"
  R0_Type/1 -> Bus Creator7/7  "R0_Type"
  R0_LC/1 -> Bus Creator7/11  "R0_LC"
  R0_VR/1 -> Bus Creator7/5  "R0_VR"
  R0_C3/1 -> Bus Creator7/4  "R0_C3"
  R0_W/1 -> Bus Creator7/9  "R0_W"
  R0_C2/1 -> Bus Creator7/3  "R0_C2"
  R0_Q/1 -> Bus Creator7/6  "R0_Q"
  R0_C0/1 -> Bus Creator7/1  "R0_C0"
  R0_TLC/1 -> Bus Creator7/10  "R0_TLC"
  R0_C1/1 -> Bus Creator7/2  "R0_C1"
  R1_C1/1 -> Bus Creator15/2  "R1_C1"
  R1_TLC/1 -> Bus Creator15/10  "R1_TLC"
  R1_C0/1 -> Bus Creator15/1  "R1_C0"
  R1_Q/1 -> Bus Creator15/6  "R1_Q"
  R1_C2/1 -> Bus Creator15/3  "R1_C2"
  R1_W/1 -> Bus Creator15/9  "R1_W"
  R1_C3/1 -> Bus Creator15/4  "R1_C3"
  R1_VR/1 -> Bus Creator15/5  "R1_VR"
  R1_LC/1 -> Bus Creator15/11  "R1_LC"
  R1_Type/1 -> Bus Creator15/7  "R1_Type"
  R1_C/1 -> Bus Creator15/8  "R1_C"
  L1_C/1 -> Bus Creator16/8  "L1_C"
  L1_Type/1 -> Bus Creator16/7  "L1_Type"
  L1_LC/1 -> Bus Creator16/11  "L1_LC"
  L1_VR/1 -> Bus Creator16/5  "L1_VR"
  L1_C3/1 -> Bus Creator16/4  "L1_C3"
  L1_W/1 -> Bus Creator16/9  "L1_W"
  L1_C2/1 -> Bus Creator16/3  "L1_C2"
  L1_Q/1 -> Bus Creator16/6  "L1_Q"
  L1_C0/1 -> Bus Creator16/1  "L1_C0"
  L1_TLC/1 -> Bus Creator16/10  "L1_TLC"
  L1_C1/1 -> Bus Creator16/2  "L1_C1"
  Bus Creator7/1 -> [bsFusR0Info]  "bsFusR0Info"
  Bus Creator16/1 -> [bsFusL1Info]  "bsFusL1Info"
  Bus Creator15/1 -> [bsFusR1Info]  "bsFusR1Info"
  Sensor_Status/1 -> Bus Creator17/1  "Sensor_Status"
  Fusion_Status/1 -> Bus Creator17/2  "Fusion_Status"
  Lane_Valid/1 -> Bus Creator17/3  "Lane_Valid"
  Road_Type/1 -> Bus Creator17/4  "Road_Type"
  ConsArea/1 -> Bus Creator17/5  "ConsArea"
  CameraSynFault/1 -> Bus Creator17/6  "CameraSynFault"
  Camera_Status/1 -> Bus Creator17/7  "Camera_Status"
  Bus Creator17/1 -> [bsFusLaneInfo]  "bsFusLaneInfo"
  O_Lane_Valid/1 -> Bus Creator18/1  "O_Lane_Valid"
  O_Lane_ConsArea/1 -> Bus Creator18/2  "O_Lane_ConsArea"
  O_Lane_RoadType/1 -> Bus Creator18/3  "O_Lane_RoadType"
  Bus Creator18/1 -> [bsOriLaneInfo]  "bsOriLaneInfo"
  O_L0_C3/1 -> Bus Creator19/1  "O_L0_C3"
  O_L0_C2/1 -> Bus Creator19/2  "O_L0_C2"
  O_L0_C1/1 -> Bus Creator19/3  "O_L0_C1"
  O_L0_C0/1 -> Bus Creator19/4  "O_L0_C0"
  O_L0_Q/1 -> Bus Creator19/5  "O_L0_Q"
  O_L0_Type/1 -> Bus Creator19/6  "O_L0_Type"
  O_L0_VR/1 -> Bus Creator19/7  "O_L0_VR"
  O_L0_TLC/1 -> Bus Creator19/8  "O_L0_TLC"
  O_L0_W/1 -> Bus Creator19/9  "O_L0_W"
  O_L0_LC/1 -> Bus Creator19/10  "O_L0_LC"
  Bus Creator19/1 -> [bsOriL0Info]  "bsOriL0Info"
  Bus Creator20/1 -> [bsOriL1Info]  "bsOriL1Info"
  O_L1_C3/1 -> Bus Creator20/1  "O_L1_C3"
  O_L1_C2/1 -> Bus Creator20/2  "O_L1_C2"
  O_L1_C1/1 -> Bus Creator20/3  "O_L1_C1"
  O_L1_C0/1 -> Bus Creator20/4  "O_L1_C0"
  O_L1_Q/1 -> Bus Creator20/5  "O_L1_Q"
  O_L1_Type/1 -> Bus Creator20/6  "O_L1_Type"
  O_L1_VR/1 -> Bus Creator20/7  "O_L1_VR"
  O_L1_TLC/1 -> Bus Creator20/8  "O_L1_TLC"
  O_L1_W/1 -> Bus Creator20/9  "O_L1_W"
  O_L1_LC/1 -> Bus Creator20/10  "O_L1_LC"
  Bus Creator22/1 -> [bsOriR1Info]  "bsOriR1Info"
  Bus Creator21/1 -> [bsOriR0Info]  "bsOriR0Info"
  O_R0_C3/1 -> Bus Creator21/1  "O_R0_C3"
  O_R0_C2/1 -> Bus Creator21/2  "O_R0_C2"
  O_R0_C1/1 -> Bus Creator21/3  "O_R0_C1"
  O_R0_C0/1 -> Bus Creator21/4  "O_R0_C0"
  O_R0_Q/1 -> Bus Creator21/5  "O_R0_Q"
  O_R0_Type/1 -> Bus Creator21/6  "O_R0_Type"
  O_R0_VR/1 -> Bus Creator21/7  "O_R0_VR"
  O_R0_TLC/1 -> Bus Creator21/8  "O_R0_TLC"
  O_R0_W/1 -> Bus Creator21/9  "O_R0_W"
  O_R0_LC/1 -> Bus Creator21/10  "O_R0_LC"
  O_R1_C2/1 -> Bus Creator22/2  "O_R1_C2"
  O_R1_C3/1 -> Bus Creator22/1  "O_R1_C3"
  O_R1_C1/1 -> Bus Creator22/3  "O_R1_C1"
  O_R1_C0/1 -> Bus Creator22/4  "O_R1_C0"
  O_R1_Q/1 -> Bus Creator22/5  "O_R1_Q"
  O_R1_Type/1 -> Bus Creator22/6  "O_R1_Type"
  O_R1_VR/1 -> Bus Creator22/7  "O_R1_VR"
  O_R1_TLC/1 -> Bus Creator22/8  "O_R1_TLC"
  O_R1_W/1 -> Bus Creator22/9  "O_R1_W"
  O_R1_LC/1 -> Bus Creator22/10  "O_R1_LC"
  Bus Creator8/1 -> [bsFusL0Info]  "bsFusL0Info"
  [bsOriLaneInfo] -> Bus Creator23/1
  [bsOriL0Info] -> Bus Creator23/2
  [bsOriL1Info] -> Bus Creator23/3
  [bsOriR0Info] -> Bus Creator23/4
  [bsOriR1Info] -> Bus Creator23/5
  [bsFusLaneInfo] -> Bus Creator23/6
  [bsFusL0Info] -> Bus Creator23/7
  [bsFusR0Info] -> Bus Creator23/8
  [bsFusL1Info] -> Bus Creator23/9
  [bsFusR1Info] -> Bus Creator23/10
  Bus Creator23/1 -> [bsLaneInfo]  "bsLaneInfo"
  Bus Creator11/1 -> [Fusion_AdditionalInf]  "Fusion_AdditionalInf"
  [Fusion_AdditionalInf] -> Bus Creator23/11
  Subsystem/1(DTC_Indicator) -> [bsDTC_Indicator]  "DTC_Indicator"
  State/1(stState) -> [bsStateInfo]  "State"
  Bus Creator5/1 -> bsInInfo/1  "bsInInfo"

== system LKAS_SIL/LL/Fault_Diagnostic ==
  bsInInfo : Inport
  Bus Creator : BusCreator  Inputs=2
  Bus Creator1 : BusCreator  Inputs=12
  Bus Selector3 : BusSelector  OutputSignals=DTC_Indicator.LKAS_BSWDTC_Status
  Bus Selector4 : BusSelector  OutputSignals=bsVehMovInfo.ESC_VehSpd_Valid,bsEPSInfo.EPS_LKA_State,bsEPSInfo.EPS_Error_State,bsEPSInfo.SAS_Clb_State,bsEPSInfo.SAS_Trim_State,bsSWAInfo.SWS_Fault_Code,bsSWAInfo.SAS_In_Status,bsPTState.TCU_ActualGear,bsEPSInfo.EPS_TrqLim_State,bsEPSInfo.EPS_Trq_State,bsVehMovInfo.ESC_LatAcc_Valid,bsVehMovInfo.ESC_YawRate_Valid,bsVehMovInfo.ESC_LonAcc_Valid
  Compare To Constant26 : simulink/Logic and Bit Operations/Compare To Constant  relop=~=  const=1  OutDataTypeStr=boolean
  Compare To Constant27 : simulink/Logic and Bit Operations/Compare To Constant  relop===  const=4  OutDataTypeStr=boolean
  Compare To Constant{28,30,36..39} (6 alike) : simulink/Logic and Bit Operations/Compare To Constant  relop===  const=1  OutDataTypeStr=boolean
  Compare To Constant29 : simulink/Logic and Bit Operations/Compare To Constant  relop===  const=0  OutDataTypeStr=boolean
  Compare To Constant31 : simulink/Logic and Bit Operations/Compare To Constant  relop===  const=2  OutDataTypeStr=boolean
  Compare To Constant32 : simulink/Logic and Bit Operations/Compare To Constant  relop=~=  const=0  OutDataTypeStr=boolean
  Compare To Constant33 : simulink/Logic and Bit Operations/Compare To Constant  relop=~=  const=1  OutDataTypeStr=boolean
  Compare To Constant34 : simulink/Logic and Bit Operations/Compare To Constant  relop=>  const=3  OutDataTypeStr=boolean
  Compare To Constant35 : simulink/Logic and Bit Operations/Compare To Constant  relop===  const=0  OutDataTypeStr=boolean
  Logical Operator5 : Logic  Operator=OR  AllPortsSameDT=off  OutDataTypeStr=boolean
  Logical Operator6 : Logic  Operator=OR  AllPortsSameDT=off  OutDataTypeStr=boolean
  bsSignalFault : Outport
  wires:
  Logical Operator6/1 -> Bus Creator1/6  "Event_FaulSWS"
  Logical Operator5/1 -> Bus Creator1/3  "Event_FaulETATDA"
  Compare To Constant27/1 -> Bus Creator1/2  "Event_FaulEPSLKASt"
  Bus Creator1/1 -> Bus Creator/2  "LKAS_ASWDTC_Status"
  Compare To Constant39/1 -> Bus Creator1/12  "Event_FaulLonAcc"
  Compare To Constant38/1 -> Bus Creator1/11  "Event_FaulYawRate"
  Compare To Constant37/1 -> Bus Creator1/10  "Event_FaulLatAcc"
  Compare To Constant36/1 -> Bus Creator1/9  "Event_FaulEPSTrqSt"
  Compare To Constant34/1 -> Bus Creator1/7  "Event_FaulTCUGear"
  Compare To Constant35/1 -> Bus Creator1/8  "Event_FaulTrqLim"
  Compare To Constant33/1 -> Logical Operator6/2
  Compare To Constant32/1 -> Logical Operator6/1
  Bus Selector4/3 -> Compare To Constant28/1, Compare To Constant31/1  "<EPS_Error_State>"
  Compare To Constant28/1 -> Logical Operator5/1
  Compare To Constant31/1 -> Logical Operator5/2
  Compare To Constant30/1 -> Bus Creator1/5  "Event_FaulSASTrim"
  Bus Selector4/13 -> Compare To Constant39/1  "<ESC_LonAcc_Valid>"
  Bus Selector4/12 -> Compare To Constant38/1  "<ESC_YawRate_Valid>"
  Bus Selector4/11 -> Compare To Constant37/1  "<ESC_LatAcc_Valid>"
  Bus Selector4/10 -> Compare To Constant36/1  "<EPS_Trq_State>"
  Bus Selector4/9 -> Compare To Constant35/1  "<EPS_TrqLim_State>"
  Bus Selector4/8 -> Compare To Constant34/1  "<TCU_ActualGear>"
  Bus Selector4/7 -> Compare To Constant33/1  "<SAS_In_Status>"
  Bus Selector4/6 -> Compare To Constant32/1  "<SWS_Fault_Code>"
  Bus Selector4/5 -> Compare To Constant30/1  "<SAS_Trim_State>"
  Compare To Constant29/1 -> Bus Creator1/4  "Event_FaulSASClb"
  Bus Selector4/4 -> Compare To Constant29/1  "<SAS_Clb_State>"
  Bus Selector4/2 -> Compare To Constant27/1  "<EPS_LKA_State>"
  Compare To Constant26/1 -> Bus Creator1/1  "Event_FaulVehSpeed"
  Bus Selector4/1 -> Compare To Constant26/1  "<ESC_VehSpd_Valid>"
  bsInInfo/1 -> Bus Selector3/1, Bus Selector4/1
  Bus Selector3/1 -> Bus Creator/1  "<LKAS_BSWDTC_Status>"
  Bus Creator/1 -> bsSignalFault/1
